simulink model "cca_scg007c"  (Simulink 9.2)
settings: Solver=FixedStepDiscrete  StartTime=0.0  StopTime=inf  FixedStep=UNIT_base_time_step  RelTol=1e-3  EnableMultiTasking=on
libraries: unit_blockset x19, unit_blockset_dataaccess x11, unit_blockset_pwm_io x2
CloseFcn:
  | rtwprivate ssgencode ModelCloseRequest Toplevel
settings Model: Creator=ajo2si  LastModifiedBy=Igor.Zanetti
settings Model: ModifiedHistory=|
  | 0.10		FST_control added
  | 0.20		ADC_control added
  | 0.21		direct mode for ADC_getValueTS implemented
  | 3.10		added block Performance Monitor
  | 3.11                    added block Syslog
  | 3.12                    new version block
settings OptimizationCC: DefaultParameterBehavior=Inlined  EnhancedBackFolding=on  ExpressionDepthLimit=2147483647  InitFltsAndDblsToZero=on  LifeSpan=Inf
settings DebuggingCC: SaveWithParameterizedLinksMsg=none  SignalResolutionControl=TryResolveAllWithWarning  SolverPrmCheckMsg=warning  MultiTaskDSMMsg=warning  MultiTaskCondExecSysMsg=none  MultiTaskRateTransMsg=warning  ParameterTunabilityLossMsg=error
settings HardwareCC: ProdLargestAtomicInteger=Long  ProdLargestAtomicFloat=Double  ProdEndianess=LittleEndian  ProdHWDeviceType=ARM Compatible->ARM 11  TargetLargestAtomicInteger=Long  TargetLargestAtomicFloat=Double  TargetIntDivRoundTo=Zero  TargetEndianess=BigEndian  TargetHWDeviceType=Freescale->MPC52xx  ProdEqTarget=off
settings SFSimCC: MATLABDynamicMemAlloc=off
settings RTWCC: SystemTargetFile=UNIT3.tlc  TemplateMakefile=UNIT3.tmf  Description=RTW Embedded Coder for UNIT3
settings CodeAppCC: IgnoreCustomStorageClasses=off  MaxIdLength=63  CustomSymbolStrType=$N$R$M  CustomSymbolStrFcn=$R$N$M$F_P3  InternalIdentifier=Classic
settings STFCustomTargetCC: UtilityFuncGeneration=Shared location  GenerateSampleERTMain=on  CombineOutputUpdateFcns=on  ERTCustomFileBanners=on  SupportContinuousTime=off  SupportNonInlinedSFcns=off  RemoveResetFunc=on  MATLABClassNameForMDSCustomization=Simulink.SoftwareTarget.ERTCustomization  GRTInterface=off  SystemTargetFile=UNIT3.tlc
settings ERTTargetCC: UtilityFuncGeneration=Shared location  MultiwordLength=2048  GenerateSampleERTMain=on  ParMdlRefBuildCompliant=off  CompOptLevelCompliant=off  ConcurrentExecutionCompliant=off  ModelStepFunctionPrototypeControlCompliant=off  CPPClassGenCompliant=off  UseToolchainInfoCompliant=off  ExtModeMexFile=noextcomm  InlinedParameterPlacement=NonHierarchical  ERTCustomFileTemplate=example_file_process.tlc  ConvertIfToSwitch=off  SuppressUnreachableDefaultCases=off

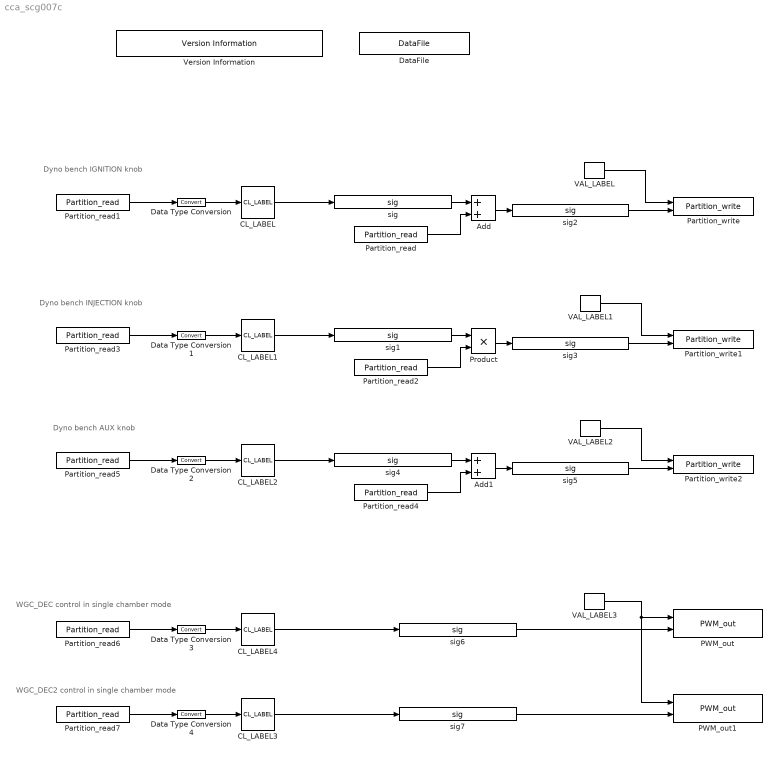
== system cca_scg007c ==
  note: Dyno bench IGNITION knob
  note: Dyno bench INJECTION knob
  note: Dyno bench AUX knob
  note: WGC_DEC control in single chamber mode
  note: WGC_DEC2 control in single chamber mode
  Add : Sum
  Add1 : Sum
  CL_LABEL : unit_blockset/DataManagement/CL_LABEL  parameter_name=MP_DIGNADDER_pod  lookup_method=Interpolation-Use End Values  outport_data_type=single  sample_time=0.001
      settings: AttributesFormatString=MP_DIGNADDER_pod
  CL_LABEL1 : unit_blockset/DataManagement/CL_LABEL  parameter_name=MP_RLPGAIN_pod  lookup_method=Interpolation-Use End Values  outport_data_type=single  sample_time=0.001
      settings: AttributesFormatString=MP_RLPGAIN_pod
  CL_LABEL2 : unit_blockset/DataManagement/CL_LABEL  parameter_name=MP_AOINJADDER_pod  lookup_method=Interpolation-Use End Values  outport_data_type=single  sample_time=0.001
      settings: AttributesFormatString=MP_AOINJADDER_pod
  CL_LABEL3 : unit_blockset/DataManagement/CL_LABEL  parameter_name=WGCDEC2PWM_pod  lookup_method=Interpolation-Use End Values  outport_data_type=single  sample_time=0.001
      settings: AttributesFormatString=WGCDEC2PWM_pod
  CL_LABEL4 : unit_blockset/DataManagement/CL_LABEL  parameter_name=WGCDECPWM_pod  lookup_method=Interpolation-Use End Values  outport_data_type=single  sample_time=0.001
      settings: AttributesFormatString=WGCDECPWM_pod
  Data Type Conversion{,1..4} (5 alike) : DataTypeConversion
  DataFile : unit_blockset/DataManagement/DataFile  filename=cca_scg007c_data.m  overwrite=on
  PWM_out : unit_blockset_pwm_io/PWM_out  ChannelName=WGC_DEC_pod  FreqValue=100  DutyValue=100  SampleTime=-1  FreqInput=0  DutyInput=0  SwitchMode=0
  PWM_out1 : unit_blockset_pwm_io/PWM_out  ChannelName=WGC_DEC2_pod  FreqValue=100  DutyValue=100  SampleTime=-1  FreqInput=0  DutyInput=0  SwitchMode=0
  Partition_read : unit_blockset_dataaccess/Partition_read  valuename=ign_map  redefine_sampletime=off  sampletime=0.1
  Partition_read1 : unit_blockset_dataaccess/Partition_read  valuename=udam_fr  redefine_sampletime=off  sampletime=0.1
  Partition_read2 : unit_blockset_dataaccess/Partition_read  valuename=rlp_map_rl  redefine_sampletime=off  sampletime=0.1
  Partition_read3 : unit_blockset_dataaccess/Partition_read  valuename=udam_fl  redefine_sampletime=off  sampletime=0.1
  Partition_read4 : unit_blockset_dataaccess/Partition_read  valuename=aoinj_map  redefine_sampletime=off  sampletime=0.1
  Partition_read5 : unit_blockset_dataaccess/Partition_read  valuename=udam_rl  redefine_sampletime=off  sampletime=0.1
  Partition_read6 : unit_blockset_dataaccess/Partition_read  valuename=wgc_pwm  redefine_sampletime=off  sampletime=0.1
  Partition_read7 : unit_blockset_dataaccess/Partition_read  valuename=wgc_pwm2  redefine_sampletime=off  sampletime=0.1
  Partition_write : unit_blockset_dataaccess/Partition_write  VariableName=ign_map  EnableInput=on
  Partition_write1 : unit_blockset_dataaccess/Partition_write  VariableName=rlp_map_rl  EnableInput=on
  Partition_write2 : unit_blockset_dataaccess/Partition_write  VariableName=aoinj_map  EnableInput=on
  Product : Product
  VAL_LABEL : unit_blockset/DataManagement/VAL_LABEL  parameter_name=CWDIGNADDEREN_pod  outport_data_type=boolean  sample_time=0.001
      settings: AttributesFormatString=%<parameter_name>
  VAL_LABEL1 : unit_blockset/DataManagement/VAL_LABEL  parameter_name=CWRLPGAINEN_pod  outport_data_type=boolean  sample_time=0.001
      settings: AttributesFormatString=%<parameter_name>
  VAL_LABEL2 : unit_blockset/DataManagement/VAL_LABEL  parameter_name=CWAOINJADDEREN_pod  outport_data_type=boolean  sample_time=0.001
      settings: AttributesFormatString=%<parameter_name>
  VAL_LABEL3 : unit_blockset/DataManagement/VAL_LABEL  parameter_name=WGC_FREQ_pod  outport_data_type=single  sample_time=0.001
      settings: AttributesFormatString=%<parameter_name>
  Version Information : unit_blockset/Version Information  Tag=UNIT_blockset_version_information  title=UNIT-Blockset Library  copyright=Copyright (c) 2013 by Bosch Engineering GmbH  compatibility=1  version=10  revision=0  annotation=cca_scg007c  state=on  program_delivery_name=Annotation field  unit_blockset_compatibility=1.194.0
  sig : unit_blockset/DataManagement/sig  signalLabel=dignadder_pod
  sig1 : unit_blockset/DataManagement/sig  signalLabel=rlpgain_pod
  sig2 : unit_blockset/DataManagement/sig  signalLabel=ign_map_pod
  sig3 : unit_blockset/DataManagement/sig  signalLabel=rlp_map_rl_pod
  sig4 : unit_blockset/DataManagement/sig  signalLabel=daoinjadder_pod
  sig5 : unit_blockset/DataManagement/sig  signalLabel=aoinj_map_pod
  sig6 : unit_blockset/DataManagement/sig  signalLabel=wgcdecpwm_pod
  sig7 : unit_blockset/DataManagement/sig  signalLabel=wgcdec2pwm_pod
  wires:
  CL_LABEL/1 -> sig/1
  sig/1 -> Add/1
  Partition_read/1 -> Add/2
  VAL_LABEL/1 -> Partition_write/1
  Add/1 -> sig2/1
  Partition_read1/1 -> Data Type Conversion/1
  Data Type Conversion/1 -> CL_LABEL/1
  CL_LABEL1/1 -> sig1/1
  Data Type Conversion1/1 -> CL_LABEL1/1
  Product/1 -> sig3/1
  VAL_LABEL1/1 -> Partition_write1/1
  Partition_read2/1 -> Product/2
  Partition_read3/1 -> Data Type Conversion1/1
  sig1/1 -> Product/1
  sig2/1 -> Partition_write/2
  sig3/1 -> Partition_write1/2
  sig5/1 -> Partition_write2/2
  sig4/1 -> Add1/1
  Partition_read5/1 -> Data Type Conversion2/1
  Partition_read4/1 -> Add1/2
  VAL_LABEL2/1 -> Partition_write2/1
  Add1/1 -> sig5/1
  Data Type Conversion2/1 -> CL_LABEL2/1
  CL_LABEL2/1 -> sig4/1
  Partition_read6/1 -> Data Type Conversion3/1
  Data Type Conversion3/1 -> CL_LABEL4/1
  Partition_read7/1 -> Data Type Conversion4/1
  Data Type Conversion4/1 -> CL_LABEL3/1
  CL_LABEL3/1 -> sig7/1
  CL_LABEL4/1 -> sig6/1
  VAL_LABEL3/1 -> PWM_out1/1, PWM_out/1
  sig6/1 -> PWM_out/2
  sig7/1 -> PWM_out1/2
